simulink model "Tetrahedron"  (R2015b)
settings: Solver=VariableStepAuto  StartTime=0.0  StopTime=10.0  RelTol=1e-3
settings Model: Creator=jn  LastModifiedBy=jn

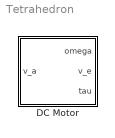
== system Tetrahedron ==
  DC Motor : Subsystem  mask{J=0.01, b=0.1, Ke=0.01, Kt=0.01, Ra=1}
      mask prompts: J "Moment of Inertia of Reaction wheel [kg*m^2]"; b "Motor Viscout friction constant [Nms]"; Ke "electromotive force constant [V/rad/sec]"; Kt "motor torque constant [Nm/Amp]"; Ra "electric resistance [Ohm]"

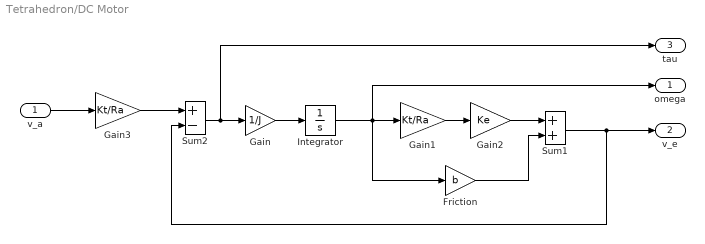
== system Tetrahedron/DC Motor ==
  v_a : Inport
  Friction : Gain  Gain=b
  Gain : Gain  Gain=1/J
  Gain1 : Gain  Gain=Kt/Ra
  Gain2 : Gain  Gain=Ke
  Gain3 : Gain  Gain=Kt/Ra
  Integrator : Integrator
  Sum1 : Sum
  Sum2 : Sum  Inputs=+-
  omega : Outport
  v_e : Outport  Port=2
  tau : Outport  Port=3
  wires:
  Sum2/1 -> tau/1, Gain/1
  Gain2/1 -> Sum1/1
  v_a/1 -> Gain3/1
  Integrator/1 -> omega/1, Friction/1, Gain1/1
  Friction/1 -> Sum1/2
  Gain3/1 -> Sum2/1
  Gain/1 -> Integrator/1
  Sum1/1 -> v_e/1, Sum2/2
  Gain1/1 -> Gain2/1
